simulink model "Kontroll_av_Heq"  (R2023b)
settings: Solver=VariableStepAuto  StartTime=0.0  StopTime=5  RelTol=1e-3
values from neighbouring files (symbols this model uses):
  D_hiv_fart = [M(3),rho_vann*Cd*A_z*Z_2]    [Overforingsfunksjon_Translasjon.m]
settings Model: Creator=anneb  LastModifiedBy=anneb

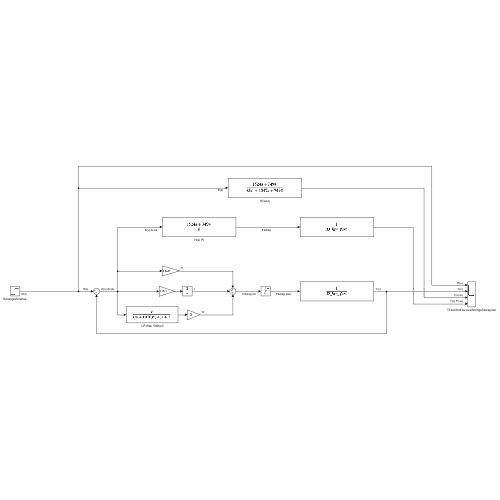
[thumbnail: Simulink's stored preview of the top-level diagram]
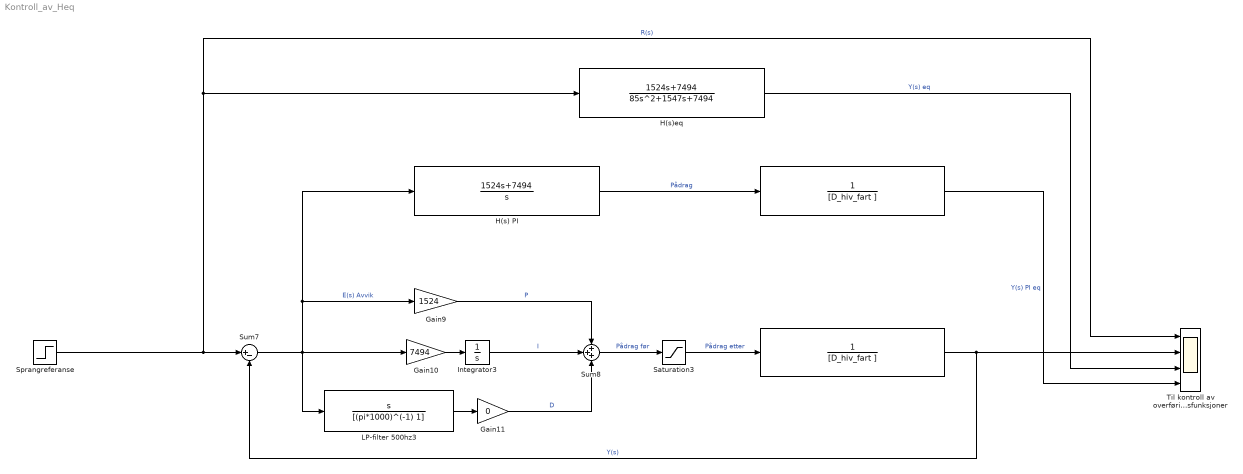
== system Kontroll_av_Heq ==
  " " : TransferFcn  Denominator=[D_hiv_fart ]
  "  " : TransferFcn  Denominator=[D_hiv_fart ]
  " LP-filter 500hz3" : TransferFcn  Numerator=[1 0]  Denominator=[(pi*1000)^(-1) 1]
  Gain10 : Gain  Gain=7494
  Gain11 : Gain  Gain=0
  Gain9 : Gain  Gain=1524
  H(s) PI : TransferFcn  Numerator=[1524 7494]  Denominator=[1 0 ]
  H(s)eq : TransferFcn  Numerator=[1524 7494]  Denominator=[85 1547 +7494 ]
  Integrator3 : Integrator
  Saturation3 : Saturate  UpperLimit=115  LowerLimit=-145
  Sprangreferanse : Step  After=0.0325  SampleTime=0
  Sum7 : Sum  Inputs=|+-
  Sum8 : Sum  Inputs=+++
  Til kontroll av overføringsfunksjoner : Scope  NumInputPorts=4
  wires:
  " "/1 -> Til kontroll av overføringsfunksjoner/4  "Y(s) PI eq"
  H(s)eq/1 -> Til kontroll av overføringsfunksjoner/3  "Y(s) eq"
  H(s) PI/1 -> " "/1  "Pådrag"
  Gain10/1 -> Integrator3/1
  "  "/1 -> Sum7/2, Til kontroll av overføringsfunksjoner/2  "Y(s)"
  Saturation3/1 -> "  "/1  "Pådrag etter"
  " LP-filter 500hz3"/1 -> Gain11/1
  Integrator3/1 -> Sum8/2  "I"
  Gain11/1 -> Sum8/3  "D"
  Sum8/1 -> Saturation3/1  "Pådrag før"
  Sprangreferanse/1 -> H(s)eq/1, Til kontroll av overføringsfunksjoner/1, Sum7/1  "R(s)"
  Gain9/1 -> Sum8/1  "P"
  Sum7/1 -> H(s) PI/1, Gain9/1, " LP-filter 500hz3"/1, Gain10/1  "E(s) Avvik"
